simulink model "Ex01"  (R2021b)
settings: Solver=VariableStepAuto  StartTime=0.0  StopTime=10.0  RelTol=1e-3
settings Model: Creator=carlo  LastModifiedBy=carlo
settings SolverCC: AlgebraicLoopSolver=TrustRegion
settings DebuggingCC: SFMachineParentedDataDiag=warning

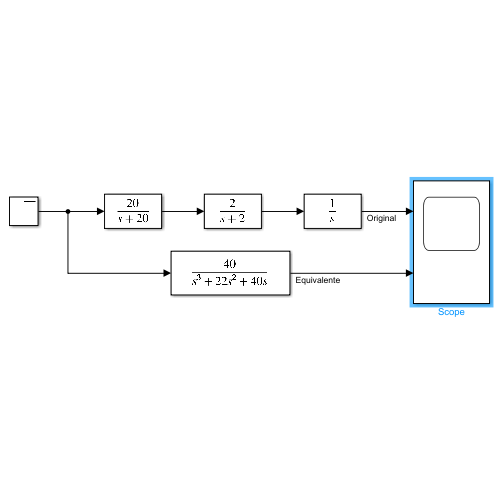
[thumbnail: Simulink's stored preview of the top-level diagram]
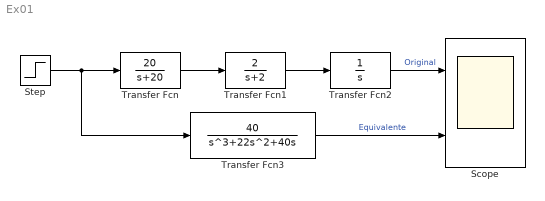
== system Ex01 ==
  Scope : Scope  NumInputPorts=2
  Step : Step  SampleTime=0
  Transfer Fcn : TransferFcn  Numerator=20  Denominator=[1 20]
  Transfer Fcn1 : TransferFcn  Numerator=2  Denominator=[1 2]
  Transfer Fcn2 : TransferFcn  Numerator=1  Denominator=[1 0]
  Transfer Fcn3 : TransferFcn  Numerator=[40]  Denominator=[1 22 40 0]
  wires:
  Transfer Fcn3/1 -> Scope/2  "Equivalente"
  Step/1 -> Transfer Fcn3/1, Transfer Fcn/1
  Transfer Fcn2/1 -> Scope/1  "Original"
  Transfer Fcn1/1 -> Transfer Fcn2/1
  Transfer Fcn/1 -> Transfer Fcn1/1
